simulink model "IFACS_Spring2026"  (R2025b)
settings: Solver=ode23t  StartTime=0.0  StopTime=3600*24*3  FixedStep=1  RelTol=1e-3  AbsTol=1e-3
values from neighbouring files (symbols this model uses):
  ac_cooling_capacity = 5000    [IFACS_Constants.m]
  ac_power = ac_cooling_capacity / ac_COP    (= 1250)    [IFACS_Constants.m]
  house_H = 6    [IFACS_Constants.m]
  house_L = 20    [IFACS_Constants.m]
  house_W = 10    [IFACS_Constants.m]
  roof_pitch = 15    [IFACS_Constants.m]
  TinIC = 24    [IFACS_Constants.m]
libraries: fl_lib x215, nesl_utility x52, simulink_extras x29, SimscapeFluids_lib x3
(part 1 of 5)
CloseFcn:
  | try,close(h1_HouseHeatingSystem),end
  | try,close(h2_HouseHeatingSystem),end
  | clear h1_HouseHeatingSystem h2_HouseHeatingSystem
  | 
  | clear simlog_HouseHeatingSystem
Description:
  | House Heating System
settings Model: FPTRunName=Active  ExtModeTrigMode=oneshot  ExtModeArmWhenConnect=off  ExtModeAutoUpdateStatusClock=off  VariantFading=off  Creator=The MathWorks, Inc.  LastModifiedBy=benir
settings SolverCC: AutoScaleAbsTol=off  MaxConsecutiveMinStep=10000  AlgebraicLoopSolver=TrustRegion
settings DataIOCC: ExternalInput=[]  InitialState=[]  SaveFormat=Array  SaveOutput=off  SaveTime=off  ReturnWorkspaceOutputs=off  SignalLoggingName=househeat_output
settings OptimizationCC: BlockReduction=off  BooleanDataType=off  ExpressionDepthLimit=2147483647.0  InitFltsAndDblsToZero=on  LifeSpan=inf  BufferReusableBoundary=off
settings DebuggingCC: AlgebraicLoopMsg=none  SaveWithParameterizedLinksMsg=none  SignalResolutionControl=TryResolveAllWithWarning  MultiTaskDSMMsg=warning  MultiTaskCondExecSysMsg=none  IntegerOverflowMsg=none  UnconnectedInputMsg=warning  UnconnectedOutputMsg=warning  UnconnectedLineMsg=warning  BusObjectLabelMismatch=none  AllowSymbolicDim=off  StateNameClashWarn=warning  PregeneratedLibrarySubsystemCodeDiagnostic=none  SFUnexpectedBacktrackingDiag=warning  SFNoUnconditionalDefaultTransitionDiag=warning  SFExecutionAtInitializationDiag=none  IntegerSaturationMsg=none  ArithmeticOperatorsInVariantConditions=warning
settings HardwareCC: ProdBitPerPointer=32.0  ProdBitPerSizeT=32.0  ProdBitPerPtrDiffT=32.0  ProdLargestAtomicFloat=None  ProdIntDivRoundTo=Undefined  ProdEndianess=Unspecified  ProdWordSize=32.0  ProdHWDeviceType=32-bit Generic  TargetUnknown=on
settings ModelReferenceCC: EnableRefExpFcnMdlSchedulingChecks=on  PropagateSignalLabelsOutOfModel=off
settings SFSimCC: SimUseLocalCustomCode=off  SimParseCustomCode=off  CustomCodeUndefinedFunction=UseInterfaceOnly
settings RTWCC: RTWUseLocalCustomCode=off  GPUComputeCapability=3.5  DLArmComputeVersion=19.05
settings CodeAppCC: StateflowObjectComments=on
settings GRTTargetCC: TargetFcnLib=ansi_tfl_tmw.mat  TargetLangStandard=C89/C90 (ANSI)  CombineOutputUpdateFcns=off  GRTInterface=on
settings ConfigComp: CovMetricSettings=dw  CovSaveCumulativeToWorkspaceVar=on  CovSaveSingleToWorkspaceVar=on  CovExternalEMLEnable=off  CovSFcnEnable=off
settings SimscapeCC: SimscapeLogType=all  SimscapeLogSimulationStatistics=on  SimscapeLogName=simlog_HouseHeatingSystem  SimscapeLogDataHistory=25000.0

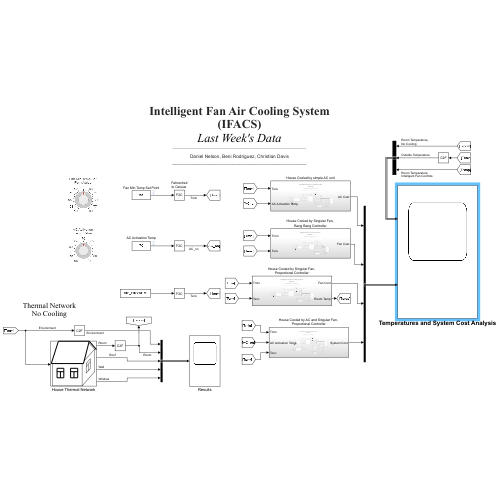
[thumbnail: Simulink's stored preview of the top-level diagram]
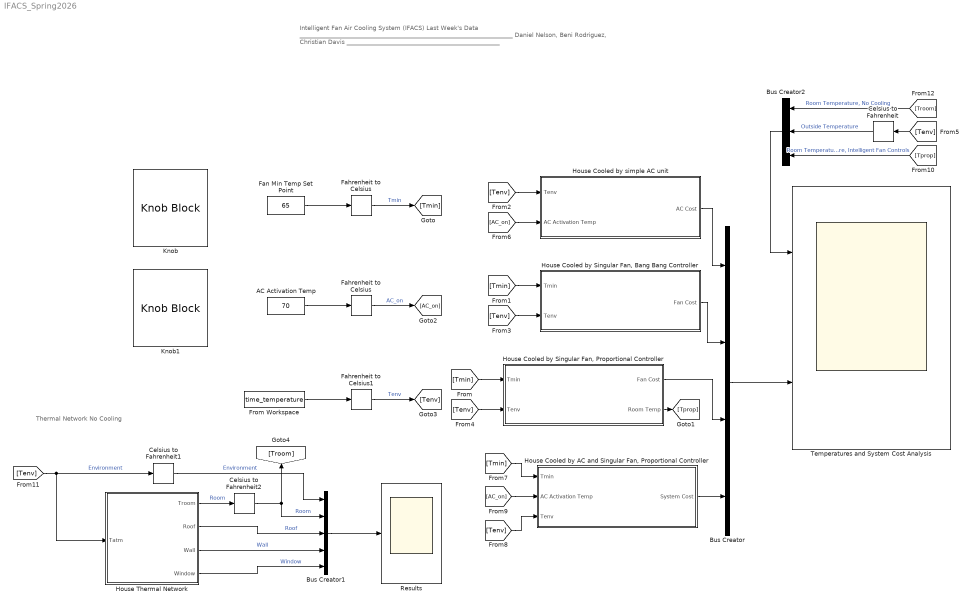
== system IFACS_Spring2026 ==
  note: Intelligent Fan Air Cooling System
      | (IFACS)
      | Last Week's Data
      | _______________________________________________________________________
      |
      | Daniel Nelson, Beni Rodriguez, Christian Davis
      | ___________________________________________________
  note: Thermal Network
      | No Cooling
  AC Activation Temp : Constant  Value=70
  Bus Creator : BusCreator  Inputs=4
  Bus Creator1 : BusCreator  Inputs=5
  Bus Creator2 : BusCreator  Inputs=3
  Celsius to Fahrenheit : simulink_extras/Transformations/Celsius to Fahrenheit
  Celsius to Fahrenheit1 : simulink_extras/Transformations/Celsius to Fahrenheit
  Celsius to Fahrenheit2 : simulink_extras/Transformations/Celsius to Fahrenheit
  Fahrenheit to Celsius : simulink_extras/Transformations/Fahrenheit to Celsius
  "Fahrenheit to Celsius " : simulink_extras/Transformations/Fahrenheit to Celsius
  Fahrenheit to Celsius1 : simulink_extras/Transformations/Fahrenheit to Celsius
  Fan Min Temp Set Point : Constant  Value=65
  From Workspace : FromWorkspace  VariableName=time_temperature
  "House Cooled by AC and Singular Fan, Proportional Controller" : Subsystem
  "House Cooled by Singular Fan, Bang Bang Controller" : Subsystem
  "House Cooled by Singular Fan, Proportional Controller" : Subsystem
  House Cooled by simple AC unit : Subsystem
  "House Thermal Network " : Subsystem  Tag=PublishSubsystem
      mask Display:
      | plot([99.4454661849886;170.309218810871;170.309218810871;99.4454661849886;99.4454661849886], [212.827470386401;212.827470386401;127.790967235342;127.790967235342;212.827470386401])
      | plot([99.4454661849886;170.309218810871], [184.481969336048;184.481969336048])
      | plot([133.460067445412;133.460067445412], [184.481969336048;127.790967235342])
      | plot([241.172971436754;312.036724062636;312.036724062636;241.172971436754;241.172971436754], [212.827470386401;212.827470386401;127.790967235342;127.790967235342;212.827470386401])
      | plot([241.172971436754;312.036724062636], [184.481969336048;184.481969336048])
      | plot([275.187572697178;275.187572697178], [184.481969336048;127.790967235342])
      | plot([113.618216710165;42.7544640842825;368.727726163343;428.253278369084], [453.764229314402;255.34572196193;255.34572196193;453.764229314402])
      | plot([428.253278369084;499.117030994967], [453.764229314402;382.900476688519])
      | plot([113.618216710165;428.253278369084], [453.764229314402;453.764229314402])
      | plot([498.86507098563;499.368991004303], [382.900476688519;382.900476688519])
      | plot([482.109730364755;496.282480889931], [382.900476688519;382.900476688519])
      | plot([482.109730364755;374.396826373413], [382.900476688519;275.187572697178])
      | plot([482.109730364755;425.418728264049], [382.900476688519;439.591478789225])
      | plot([56.927214609459;56.927214609459;354.554975638166], [255.34572196193;56.927214609459;56.927214609459])
      | plot([354.554975638166;354.554975638166], [56.927214609459;255.34572196193])
      | plot([354.554975638166;482.109730364755;482.109730364755], [56.927214609459;184.481969336048;382.900476688519])
      | plot([397.073227213696;397.073227213696;439.591478789225;439.591478789225;397.073227213696], [170.309218810871;255.34572196193;297.86397353746;209.992920281366;170.309218810871])
      | plot([397.073227213696;439.591478789225], [227.000220911577;269.518472487107])
      | plot([419.749628053978;419.749628053978], [246.842071646824;192.985619651154])
      | %patch([0;553.20969549939;553.20969549939;0;0;0.472425017505884;0.47242501750577;552.737270481884;552.737270481885;0.472425017505884;0], [496.518693398684;496.518693398684;0;0;496.518693398684;496.046268381178;0.472425017505884;0.472425017505884;496.046268381178;496.046268381178;496.518693398684], [1;1;1])
  Knob : KnobBlock  ScaleMin=50  ScaleMax=80
  Knob1 : KnobBlock  ScaleMin=50  ScaleMax=90
  Results : Scope
      settings: TimeUnits=Metric (based on Time Span)  Title=Daily Room Temp  ActiveDisplayYMinimum=61.662880384493235  ActiveDisplayYMaximum=74.086551143430853  YLabel=Temperature (F)  DataLoggingVariableName=a  DataLoggingSaveFormat=Array
  Temperatures and System Cost Analysis : Scope  NumInputPorts=2
      settings: TimeUnits=Metric (based on Time Span)  Title=Temperature  ActiveDisplayYMinimum=51.858630285523695  ActiveDisplayYMaximum=88.349041079386282  YLabel=Temperature (F)
  wires:
  Fan Min Temp Set Point/1 -> "Fahrenheit to Celsius "/1
  "Fahrenheit to Celsius "/1 -> [Tmin]  "Tmin"
  [Tenv] -> House Cooled by simple AC unit/1(Tenv)
  [Tmin] -> "House Cooled by Singular Fan, Bang Bang Controller"/1(Tmin)
  [Tenv] -> "House Cooled by Singular Fan, Bang Bang Controller"/2(Tenv)
  "House Cooled by Singular Fan, Proportional Controller"/1(Fan Cost) -> Bus Creator/3
  "House Cooled by Singular Fan, Bang Bang Controller"/1(Fan Cost) -> Bus Creator/2
  House Cooled by simple AC unit/1(AC Cost) -> Bus Creator/1
  [Tenv] -> Celsius to Fahrenheit/1
  AC Activation Temp/1 -> Fahrenheit to Celsius/1
  Fahrenheit to Celsius/1 -> [AC_on]  "AC_on"
  [AC_on] -> House Cooled by simple AC unit/2(AC Activation Temp)
  From Workspace/1 -> Fahrenheit to Celsius1/1
  [Tmin] -> "House Cooled by AC and Singular Fan, Proportional Controller"/1(Tmin)
  [Tenv] -> "House Cooled by AC and Singular Fan, Proportional Controller"/3(Tenv)
  [AC_on] -> "House Cooled by AC and Singular Fan, Proportional Controller"/2(AC Activation Temp)
  "House Cooled by AC and Singular Fan, Proportional Controller"/1(System Cost) -> Bus Creator/4
  Fahrenheit to Celsius1/1 -> [Tenv]  "Tenv"
  Bus Creator/1 -> Temperatures and System Cost Analysis/2
  [Tprop] -> Bus Creator2/3  "Room Temperature, Intelligent Fan Controls"
  Celsius to Fahrenheit/1 -> Bus Creator2/2  "Outside Temperature"
  Bus Creator2/1 -> Temperatures and System Cost Analysis/1
  "House Cooled by Singular Fan, Proportional Controller"/2(Room Temp) -> [Tprop]
  [Tmin] -> "House Cooled by Singular Fan, Proportional Controller"/1(Tmin)
  [Tenv] -> "House Cooled by Singular Fan, Proportional Controller"/2(Tenv)
  "House Thermal Network "/4(Window) -> Bus Creator1/5  "Window"
  "House Thermal Network "/3(Wall) -> Bus Creator1/4  "Wall"
  Celsius to Fahrenheit1/1 -> Bus Creator1/1  "Environment"
  Bus Creator1/1 -> Results/1
  "House Thermal Network "/1(Troom) -> Celsius to Fahrenheit2/1  "Room"
  "House Thermal Network "/2(Roof) -> Bus Creator1/3  "Roof"
  [Tenv] -> "House Thermal Network "/1(Tatm), Celsius to Fahrenheit1/1  "Environment"
  Celsius to Fahrenheit2/1 -> [Troom], Bus Creator1/2  "Room"
  [Troom] -> Bus Creator2/1  "Room Temperature, No Cooling"

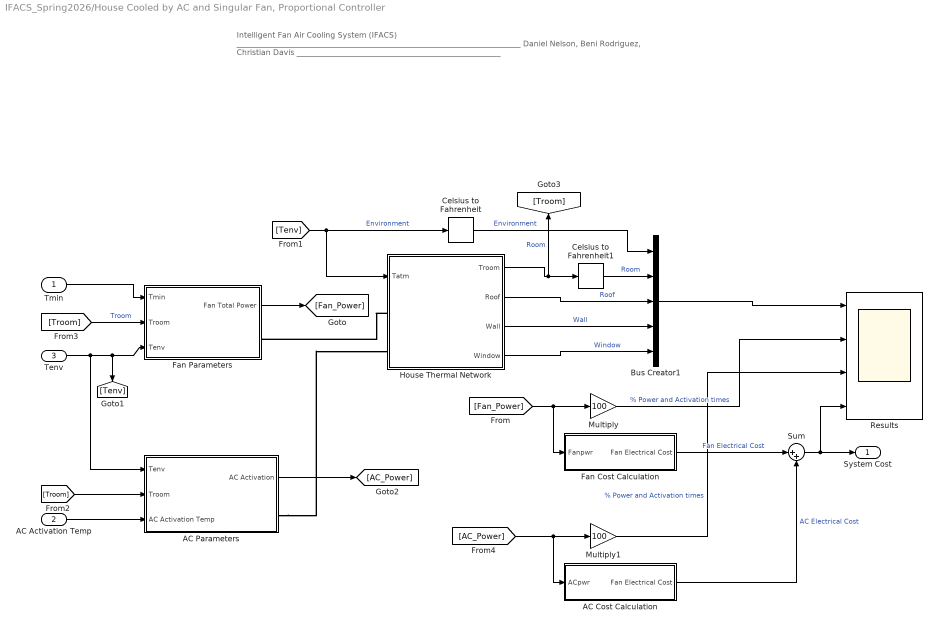
== system IFACS_Spring2026/House Cooled by AC and Singular Fan, Proportional Controller ==
  note: Intelligent Fan Air Cooling System
      | (IFACS)
      | _______________________________________________________________________
      |
      | Daniel Nelson, Beni Rodriguez, Christian Davis
      | ___________________________________________________
  Tmin : Inport
  AC Activation Temp : Inport  Port=2
  Tenv : Inport  Port=3
  AC Cost Calculation : Subsystem
  AC Parameters : Subsystem
  Bus Creator1 : BusCreator  Inputs=5
  Celsius to Fahrenheit : simulink_extras/Transformations/Celsius to Fahrenheit
  Celsius to Fahrenheit1 : simulink_extras/Transformations/Celsius to Fahrenheit
  Fan Cost Calculation : Subsystem
  Fan Parameters : Subsystem
  House Thermal Network : Subsystem  Tag=PublishSubsystem
      mask Display:
      | plot([99.4454661849886;170.309218810871;170.309218810871;99.4454661849886;99.4454661849886], [212.827470386401;212.827470386401;127.790967235342;127.790967235342;212.827470386401])
      | plot([99.4454661849886;170.309218810871], [184.481969336048;184.481969336048])
      | plot([133.460067445412;133.460067445412], [184.481969336048;127.790967235342])
      | plot([241.172971436754;312.036724062636;312.036724062636;241.172971436754;241.172971436754], [212.827470386401;212.827470386401;127.790967235342;127.790967235342;212.827470386401])
      | plot([241.172971436754;312.036724062636], [184.481969336048;184.481969336048])
      | plot([275.187572697178;275.187572697178], [184.481969336048;127.790967235342])
      | plot([113.618216710165;42.7544640842825;368.727726163343;428.253278369084], [453.764229314402;255.34572196193;255.34572196193;453.764229314402])
      | plot([428.253278369084;499.117030994967], [453.764229314402;382.900476688519])
      | plot([113.618216710165;428.253278369084], [453.764229314402;453.764229314402])
      | plot([498.86507098563;499.368991004303], [382.900476688519;382.900476688519])
      | plot([482.109730364755;496.282480889931], [382.900476688519;382.900476688519])
      | plot([482.109730364755;374.396826373413], [382.900476688519;275.187572697178])
      | plot([482.109730364755;425.418728264049], [382.900476688519;439.591478789225])
      | plot([56.927214609459;56.927214609459;354.554975638166], [255.34572196193;56.927214609459;56.927214609459])
      | plot([354.554975638166;354.554975638166], [56.927214609459;255.34572196193])
      | plot([354.554975638166;482.109730364755;482.109730364755], [56.927214609459;184.481969336048;382.900476688519])
      | plot([397.073227213696;397.073227213696;439.591478789225;439.591478789225;397.073227213696], [170.309218810871;255.34572196193;297.86397353746;209.992920281366;170.309218810871])
      | plot([397.073227213696;439.591478789225], [227.000220911577;269.518472487107])
      | plot([419.749628053978;419.749628053978], [246.842071646824;192.985619651154])
      | %patch([0;553.20969549939;553.20969549939;0;0;0.472425017505884;0.47242501750577;552.737270481884;552.737270481885;0.472425017505884;0], [496.518693398684;496.518693398684;0;0;496.518693398684;496.046268381178;0.472425017505884;0.472425017505884;496.046268381178;496.046268381178;496.518693398684], [1;1;1])
  Multiply : Gain  Gain=100
  Multiply1 : Gain  Gain=100
  Results : Scope  NumInputPorts=4
      settings: TimeUnits=Metric (based on Time Span)  ActiveDisplayString=4  Title=Total System Cost  ActiveDisplayYMinimum=-0.28869506365036945  ActiveDisplayYMaximum=5.4852062093570213  YLabel=System Cost ($)  DataLoggingVariableName=a3  DataLoggingSaveFormat=Array
  Sum : Sum  Inputs=|++
  System Cost : Outport
  wires:
  Bus Creator1/1 -> Results/1
  [Tenv] -> House Thermal Network/1(Tatm), Celsius to Fahrenheit/1  "Environment"
  House Thermal Network/1(Troom) -> Celsius to Fahrenheit1/1, [Troom]  "Room"
  Multiply/1 -> Results/2  "% Power and Activation times"
  House Thermal Network/2(Roof) -> Bus Creator1/3  "Roof"
  House Thermal Network/3(Wall) -> Bus Creator1/4  "Wall"
  House Thermal Network/4(Window) -> Bus Creator1/5  "Window"
  Tenv/1 -> AC Parameters/1(Tenv), Fan Parameters/3(Tenv), [Tenv]
  [Fan_Power] -> Fan Cost Calculation/1(Fanpwr), Multiply/1
  Celsius to Fahrenheit1/1 -> Bus Creator1/2  "Room"
  Celsius to Fahrenheit/1 -> Bus Creator1/1  "Environment"
  Tmin/1 -> Fan Parameters/1(Tmin)
  [Troom] -> Fan Parameters/2(Troom)  "Troom"
  Fan Parameters/1(Fan Total Power) -> [Fan_Power]
  Fan Cost Calculation/1(Fan Electrical Cost) -> Sum/1  "Fan Electrical Cost"
  AC Activation Temp/1 -> AC Parameters/3(AC Activation Temp)
  [Troom] -> AC Parameters/2(Troom)
  Multiply1/1 -> Results/3  "% Power and Activation times"
  AC Cost Calculation/1(Fan Electrical Cost) -> Sum/2  "AC Electrical Cost"
  [AC_Power] -> AC Cost Calculation/1(ACpwr), Multiply1/1
  Sum/1 -> Results/4, System Cost/1
  AC Parameters/1(AC Activation) -> [AC_Power]
  connections:
  House Thermal Network/LConn1 -- Fan Parameters/RConn1
  AC Parameters/RConn1 -- House Thermal Network/LConn2

== system IFACS_Spring2026/House Cooled by Singular Fan, Bang Bang Controller ==
  note: Intelligent Fan Air Cooling System
      | (IFACS)
      | _______________________________________________________________________
      |
      | Daniel Nelson, Beni Rodriguez, Christian Davis
      | ___________________________________________________
  Tmin : Inport
  Tenv : Inport  Port=2
  Bus Creator1 : BusCreator  Inputs=5
  Celsius to Fahrenheit : simulink_extras/Transformations/Celsius to Fahrenheit
  Celsius to Fahrenheit1 : simulink_extras/Transformations/Celsius to Fahrenheit
  Fan Cost Calculation : Subsystem
  Fan Parameters : Subsystem
  House Thermal Network : Subsystem  Tag=PublishSubsystem
      mask Display:
      | plot([99.4454661849886;170.309218810871;170.309218810871;99.4454661849886;99.4454661849886], [212.827470386401;212.827470386401;127.790967235342;127.790967235342;212.827470386401])
      | plot([99.4454661849886;170.309218810871], [184.481969336048;184.481969336048])
      | plot([133.460067445412;133.460067445412], [184.481969336048;127.790967235342])
      | plot([241.172971436754;312.036724062636;312.036724062636;241.172971436754;241.172971436754], [212.827470386401;212.827470386401;127.790967235342;127.790967235342;212.827470386401])
      | plot([241.172971436754;312.036724062636], [184.481969336048;184.481969336048])
      | plot([275.187572697178;275.187572697178], [184.481969336048;127.790967235342])
      | plot([113.618216710165;42.7544640842825;368.727726163343;428.253278369084], [453.764229314402;255.34572196193;255.34572196193;453.764229314402])
      | plot([428.253278369084;499.117030994967], [453.764229314402;382.900476688519])
      | plot([113.618216710165;428.253278369084], [453.764229314402;453.764229314402])
      | plot([498.86507098563;499.368991004303], [382.900476688519;382.900476688519])
      | plot([482.109730364755;496.282480889931], [382.900476688519;382.900476688519])
      | plot([482.109730364755;374.396826373413], [382.900476688519;275.187572697178])
      | plot([482.109730364755;425.418728264049], [382.900476688519;439.591478789225])
      | plot([56.927214609459;56.927214609459;354.554975638166], [255.34572196193;56.927214609459;56.927214609459])
      | plot([354.554975638166;354.554975638166], [56.927214609459;255.34572196193])
      | plot([354.554975638166;482.109730364755;482.109730364755], [56.927214609459;184.481969336048;382.900476688519])
      | plot([397.073227213696;397.073227213696;439.591478789225;439.591478789225;397.073227213696], [170.309218810871;255.34572196193;297.86397353746;209.992920281366;170.309218810871])
      | plot([397.073227213696;439.591478789225], [227.000220911577;269.518472487107])
      | plot([419.749628053978;419.749628053978], [246.842071646824;192.985619651154])
      | %patch([0;553.20969549939;553.20969549939;0;0;0.472425017505884;0.47242501750577;552.737270481884;552.737270481885;0.472425017505884;0], [496.518693398684;496.518693398684;0;0;496.518693398684;496.046268381178;0.472425017505884;0.472425017505884;496.046268381178;496.046268381178;496.518693398684], [1;1;1])
  Multiply : Gain  Gain=100
  Results : Scope  NumInputPorts=3
      settings: TimeUnits=Metric (based on Time Span)  ActiveDisplayString=3  Title=Fan Cost  ActiveDisplayYMinimum=-0.053943140725414111  ActiveDisplayYMaximum=0.48548826652872712  YLabel=Fan Cost ($)  DataLoggingVariableName=a3  DataLoggingSaveFormat=Array
  Fan Cost : Outport
  wires:
  Bus Creator1/1 -> Results/1
  [Tenv] -> House Thermal Network/1(Tatm), Celsius to Fahrenheit/1  "Environment"
  House Thermal Network/1(Troom) -> Celsius to Fahrenheit1/1, [Troom]  "Room"
  Multiply/1 -> Results/2  "% Power and Activation times"
  House Thermal Network/3(Wall) -> Bus Creator1/4  "Wall"
  House Thermal Network/4(Window) -> Bus Creator1/5  "Window"
  Tenv/1 -> Fan Parameters/3(Tenv), [Tenv]
  [Fan_Power] -> Fan Cost Calculation/1(Fanpwr), Multiply/1
  Celsius to Fahrenheit1/1 -> Bus Creator1/2  "Room"
  Celsius to Fahrenheit/1 -> Bus Creator1/1  "Environment"
  Tmin/1 -> Fan Parameters/1(Tmin)
  [Troom] -> Fan Parameters/2(Troom)  "Troom"
  Fan Parameters/1(Fan Total Power) -> [Fan_Power]
  House Thermal Network/2(Roof) -> Bus Creator1/3  "Roof"
  Fan Cost Calculation/1(Fan Electrical Cost) -> Results/3, Fan Cost/1  "Fan Electrical Cost"
  connections:
  House Thermal Network/LConn1 -- Fan Parameters/RConn1

== system IFACS_Spring2026/House Cooled by Singular Fan, Proportional Controller ==
  note: Intelligent Fan Air Cooling System
      | (IFACS)
      | _______________________________________________________________________
      |
      | Daniel Nelson, Beni Rodriguez, Christian Davis
      | ___________________________________________________
  Tmin : Inport
  Tenv : Inport  Port=2
  Bus Creator1 : BusCreator  Inputs=5
  Celsius to Fahrenheit : simulink_extras/Transformations/Celsius to Fahrenheit
  Celsius to Fahrenheit1 : simulink_extras/Transformations/Celsius to Fahrenheit
  Fan Cost Calculation : Subsystem
  Fan Parameters : Subsystem
  House Thermal Network : Subsystem  Tag=PublishSubsystem
      mask Display:
      | plot([99.4454661849886;170.309218810871;170.309218810871;99.4454661849886;99.4454661849886], [212.827470386401;212.827470386401;127.790967235342;127.790967235342;212.827470386401])
      | plot([99.4454661849886;170.309218810871], [184.481969336048;184.481969336048])
      | plot([133.460067445412;133.460067445412], [184.481969336048;127.790967235342])
      | plot([241.172971436754;312.036724062636;312.036724062636;241.172971436754;241.172971436754], [212.827470386401;212.827470386401;127.790967235342;127.790967235342;212.827470386401])
      | plot([241.172971436754;312.036724062636], [184.481969336048;184.481969336048])
      | plot([275.187572697178;275.187572697178], [184.481969336048;127.790967235342])
      | plot([113.618216710165;42.7544640842825;368.727726163343;428.253278369084], [453.764229314402;255.34572196193;255.34572196193;453.764229314402])
      | plot([428.253278369084;499.117030994967], [453.764229314402;382.900476688519])
      | plot([113.618216710165;428.253278369084], [453.764229314402;453.764229314402])
      | plot([498.86507098563;499.368991004303], [382.900476688519;382.900476688519])
      | plot([482.109730364755;496.282480889931], [382.900476688519;382.900476688519])
      | plot([482.109730364755;374.396826373413], [382.900476688519;275.187572697178])
      | plot([482.109730364755;425.418728264049], [382.900476688519;439.591478789225])
      | plot([56.927214609459;56.927214609459;354.554975638166], [255.34572196193;56.927214609459;56.927214609459])
      | plot([354.554975638166;354.554975638166], [56.927214609459;255.34572196193])
      | plot([354.554975638166;482.109730364755;482.109730364755], [56.927214609459;184.481969336048;382.900476688519])
      | plot([397.073227213696;397.073227213696;439.591478789225;439.591478789225;397.073227213696], [170.309218810871;255.34572196193;297.86397353746;209.992920281366;170.309218810871])
      | plot([397.073227213696;439.591478789225], [227.000220911577;269.518472487107])
      | plot([419.749628053978;419.749628053978], [246.842071646824;192.985619651154])
      | %patch([0;553.20969549939;553.20969549939;0;0;0.472425017505884;0.47242501750577;552.737270481884;552.737270481885;0.472425017505884;0], [496.518693398684;496.518693398684;0;0;496.518693398684;496.046268381178;0.472425017505884;0.472425017505884;496.046268381178;496.046268381178;496.518693398684], [1;1;1])
  Multiply : Gain  Gain=100
  Results : Scope  NumInputPorts=3
      settings: TimeUnits=Metric (based on Time Span)  Title=Fan Power  ActiveDisplayYMinimum=-11.770479028172618  ActiveDisplayYMaximum=105.93431125355357  YLabel=Fan Power (%)  DataLoggingVariableName=a3  DataLoggingSaveFormat=Array
  Fan Cost : Outport
  Room Temp : Outport  Port=2
  wires:
  Bus Creator1/1 -> Results/1
  [Tenv] -> House Thermal Network/1(Tatm), Celsius to Fahrenheit/1  "Environment"
  House Thermal Network/1(Troom) -> Celsius to Fahrenheit1/1, [Troom]  "Room"
  Multiply/1 -> Results/2  "% Power and Activation times"
  House Thermal Network/2(Roof) -> Bus Creator1/3  "Roof"
  House Thermal Network/3(Wall) -> Bus Creator1/4  "Wall"
  House Thermal Network/4(Window) -> Bus Creator1/5  "Window"
  Tenv/1 -> Fan Parameters/3(Tenv), [Tenv]
  [Fan_Power] -> Fan Cost Calculation/1(Fanpwr), Multiply/1
  Celsius to Fahrenheit1/1 -> Room Temp/1, Bus Creator1/2  "Room"
  Celsius to Fahrenheit/1 -> Bus Creator1/1  "Environment"
  Tmin/1 -> Fan Parameters/1(Tmin)
  [Troom] -> Fan Parameters/2(Troom)  "Troom"
  Fan Parameters/1(Fan Total Power) -> [Fan_Power]
  Fan Cost Calculation/1(Fan Electrical Cost) -> Results/3, Fan Cost/1  "Fan Electrical Cost"
  connections:
  House Thermal Network/LConn1 -- Fan Parameters/RConn1

== system IFACS_Spring2026/House Cooled by simple AC unit ==
  note: Intelligent Fan Air Cooling System
      | (IFACS)
      | _______________________________________________________________________
      |
      | Daniel Nelson, Beni Rodriguez, Christian Davis
      | ___________________________________________________
  Tenv : Inport
  AC Activation Temp : Inport  Port=2
  AC Cost Calculation : Subsystem
  AC Parameters : Subsystem
  Bus Creator1 : BusCreator  Inputs=5
  Celsius to Fahrenheit : simulink_extras/Transformations/Celsius to Fahrenheit
  Celsius to Fahrenheit1 : simulink_extras/Transformations/Celsius to Fahrenheit
  House Thermal Network : Subsystem  Tag=PublishSubsystem
      mask Display:
      | plot([99.4454661849886;170.309218810871;170.309218810871;99.4454661849886;99.4454661849886], [212.827470386401;212.827470386401;127.790967235342;127.790967235342;212.827470386401])
      | plot([99.4454661849886;170.309218810871], [184.481969336048;184.481969336048])
      | plot([133.460067445412;133.460067445412], [184.481969336048;127.790967235342])
      | plot([241.172971436754;312.036724062636;312.036724062636;241.172971436754;241.172971436754], [212.827470386401;212.827470386401;127.790967235342;127.790967235342;212.827470386401])
      | plot([241.172971436754;312.036724062636], [184.481969336048;184.481969336048])
      | plot([275.187572697178;275.187572697178], [184.481969336048;127.790967235342])
      | plot([113.618216710165;42.7544640842825;368.727726163343;428.253278369084], [453.764229314402;255.34572196193;255.34572196193;453.764229314402])
      | plot([428.253278369084;499.117030994967], [453.764229314402;382.900476688519])
      | plot([113.618216710165;428.253278369084], [453.764229314402;453.764229314402])
      | plot([498.86507098563;499.368991004303], [382.900476688519;382.900476688519])
      | plot([482.109730364755;496.282480889931], [382.900476688519;382.900476688519])
      | plot([482.109730364755;374.396826373413], [382.900476688519;275.187572697178])
      | plot([482.109730364755;425.418728264049], [382.900476688519;439.591478789225])
      | plot([56.927214609459;56.927214609459;354.554975638166], [255.34572196193;56.927214609459;56.927214609459])
      | plot([354.554975638166;354.554975638166], [56.927214609459;255.34572196193])
      | plot([354.554975638166;482.109730364755;482.109730364755], [56.927214609459;184.481969336048;382.900476688519])
      | plot([397.073227213696;397.073227213696;439.591478789225;439.591478789225;397.073227213696], [170.309218810871;255.34572196193;297.86397353746;209.992920281366;170.309218810871])
      | plot([397.073227213696;439.591478789225], [227.000220911577;269.518472487107])
      | plot([419.749628053978;419.749628053978], [246.842071646824;192.985619651154])
      | %patch([0;553.20969549939;553.20969549939;0;0;0.472425017505884;0.47242501750577;552.737270481884;552.737270481885;0.472425017505884;0], [496.518693398684;496.518693398684;0;0;496.518693398684;496.046268381178;0.472425017505884;0.472425017505884;496.046268381178;496.046268381178;496.518693398684], [1;1;1])
  Multiply : Gain  Gain=100
  Results : Scope  NumInputPorts=3
      settings: TimeUnits=Metric (based on Time Span)  ActiveDisplayString=3  ActiveDisplayYMinimum=-0.20049406109345627  ActiveDisplayYMaximum=1.8044465498411069  YLabel=AC Cost ($)  DataLoggingVariableName=a3  DataLoggingSaveFormat=Array
  AC Cost : Outport
  wires:
  Bus Creator1/1 -> Results/1
  [Tenv] -> House Thermal Network/1(Tatm), Celsius to Fahrenheit/1  "Environment"
  House Thermal Network/1(Troom) -> Celsius to Fahrenheit1/1, [Troom]  "Room"
  Multiply/1 -> Results/2  "% Power and Activation times"
  House Thermal Network/2(Roof) -> Bus Creator1/3  "Roof"
  House Thermal Network/3(Wall) -> Bus Creator1/4  "Wall"
  House Thermal Network/4(Window) -> Bus Creator1/5  "Window"
  Tenv/1 -> AC Parameters/3(Tenv), [Tenv]
  [AC_Power] -> AC Cost Calculation/1(ACpwr), Multiply/1
  Celsius to Fahrenheit1/1 -> Bus Creator1/2  "Room"
  Celsius to Fahrenheit/1 -> Bus Creator1/1  "Environment"
  [Troom] -> AC Parameters/1(Troom)  "Troom"
  AC Parameters/1(AC Activation) -> [AC_Power]
  AC Cost Calculation/1(Fan Electrical Cost) -> Results/3, AC Cost/1  "AC Electrical Cost"
  AC Activation Temp/1 -> AC Parameters/2(AC Activation Temp)
  connections:
  House Thermal Network/LConn1 -- AC Parameters/RConn1

== system IFACS_Spring2026/House Thermal Network  ==
  Tatm : Inport
  Controlled Temperature Source : fl_lib/Thermal/Thermal Sources/Controlled Temperature Source
  House Thermal Network : Subsystem  Tag=PublishSubsystem  mask(House Thermal Network){area_roof=2 * house_L * house_W / (2*cosd(roof_pitch)), thickness_roof=0.2, rho_roof=32, cp_roof=835, k_roof=0.038, hc_roof_interior=12, hc_roof_exterior=38, T_init_roof=TinIC, area_wall=2 * (house_L + house_W) * house_H, thickness_wall=0.2, rho_wall=1920, cp_wall=835, k_wall=0.038, hc_wall_interior=24, hc_wall_exterior=34, T_init_wall=TinIC, area_wall_inside=(house_L + 2 * house_W) * house_H + 2 * house_L * house_W, thickness_wall_inside=0.15, rho_wall_inside=10, cp_wall_inside=1000, k_wall_inside=0.2, hc_wall_inside_interior=24, T_init_wall_inside=TinIC, area_window=12, thickness_window=0.01, rho_window=2700, cp_window=840, k_window=0.78, hc_window_interior=25, hc_window_exterior=32, T_init_window=TinIC, area_furniture=300, M_furniture=3000, cp_furniture=2000, hc_furniture_interior=18, T_init_furniture=TinIC}
      mask prompts: area_roof "Total area (m^2)"; thickness_roof "Average thickness (m)"; rho_roof "Average density (kg/m^3)"; cp_roof "Average specific heat (J/kg/K)"; k_roof "Average conductivity (W/m/K)"; hc_roof_interior "Interior heat transfer coefficient (W/m^2/K)"; hc_roof_exterior "Exterior heat transfer coefficient (W/m^2/K)"; T_init_roof "Initial temperature (degC)"; area_wall "Total area (m^2)"; thickness_wall "Average thickness (m)"; rho_wall "Average density (kg/m^3)"; cp_wall "Average specific heat (J/kg/K)"; k_wall "Average conductivity (W/m/K)"; hc_wall_interior "Interior heat transfer coefficient (W/m^2/K)"; hc_wall_exterior "Exterior heat transfer coefficient (W/m^2/K)"; T_init_wall "Initial temperature (degC)"; area_wall_inside "Total area (m^2)"; thickness_wall_inside "Average thickness (m)"; rho_wall_inside "Average density (kg/m^3)"; cp_wall_inside "Average specific heat (J/kg/K)"; k_wall_inside "Average conductivity (W/m/K)"; hc_wall_inside_interior "Interior heat transfer coefficient (W/m^2/K)"; T_init_wall_inside "Initial temperature (degC)"; area_window "Total area (m^2)"; thickness_window "Average thickness (m)"; rho_window "Average density (kg/m^3)"; cp_window "Average specific heat (J/kg/K)"; k_window "Average conductivity (W/m/K)"; hc_window_interior "Interior heat transfer coefficient (W/m^2/K)"; hc_window_exterior "Exterior heat transfer coefficient (W/m^2/K)"; T_init_window "Initial temperature (degC)"; area_furniture "Total surface area (m^2)"; M_furniture "Total mass (kg)"; cp_furniture "Average specific heat (J/kg/K)"; hc_furniture_interior "Interior heat transfer coefficient (W/m^2/K)"; T_init_furniture "Initial temperature (degC)"
      mask help: This subsystem models heat transfer between the air in the interior of the house and the external environment.
      mask DialogControl TabRoof Prompt: Roof
      mask DialogControl TabWall Prompt: Exterior Walls
      mask DialogControl TabWallInside Prompt: Interior Walls
      mask DialogControl TabWindow Prompt: Windows
      mask DialogControl TabFurniture Prompt: Furniture
  PS2S : nesl_utility/PS-Simulink Converter  PhysicalDomain=network_engine_domain  SubClassName=ps_output  LeftPortType=input  RightPortType=output  PseudoPeriodic=off  Frequencies=[]  VectorFormat=1-D array  Unit=degC  AffineConversion=on
  Simulink-PS Converter : nesl_utility/Simulink-PS Converter  PhysicalDomain=network_engine_domain  SubClassName=ps_input  LeftPortType=input  RightPortType=output  PseudoPeriodic=off  Frequencies=[]  NoiseDistribution=none  NoiseParameters=[]  Unit=degC  AffineConversion=on  FilteringAndDerivatives=zero  SimscapeFilterOrder=1  InputFilterTimeConstant=.001  UdotUserProvided=0
  Solver Configuration : nesl_utility/Solver Configuration  PhysicalDomain=network_engine_domain  SubClassName=solver  LeftPortType=input  RightPortType=generic  Tones=[]  Harmonics=[]  SimulateNoise=off  Profile=off  UseLocalSampling=off  EnableSwitchedLinearOptims=on  FrequencyDomain=off  UseCCode=off  RelTol=0.001  AbsTol=1e-06  MinStep=1e-09  ToWorkspace=off  RevertToSquareIcSolve=off  NumHomotopyIterations=100  PhasorMode=off  PhasorModeNumHarmonics=1  ConsistencySolver=NEWTON_XTOL_AFTER_FTOL  IndexReductionMethod=DerivativeReplacement  DoDC=off  ResidualTolerance=1e-9  ConsistencyTolSource=GLOBAL  ConsistencyAbsTol=0.001  ConsistencyRelTol=0.001  ConsistencyTolFactor=0.001  UseLocalSolver=off  LocalSolverChoice=NE_BACKWARD_EULER_ADVANCER  ResolveIndetEquations=on  FunctionEvalNumThread=1  LocalSolverSampleTime=1  DoFixedCost=off  MaxNonlinIter=3  MaxModeIter=2  ComputeImpulses=off  ImpulseIterations=2  LinearAlgebra=auto  LinearAlgebraNumThread=0  EquationFormulation=NE_TIME_EF  DelaysMemoryBudget=1024  AutomaticFiltering=on  FilteringTimeConstant=0.001  PartitionStorageMethod=AS_NEEDED  PartitionMemoryBudget=1024  PartitionMethod=FAST  MultibodyUseLocalSolver=off  MultibodyLocalSolverChoice=ODE1  MultibodyLocalSolverSampleTime=0.001
  TRef : fl_lib/Thermal/Thermal Elements/Thermal Reference
  Temperature Sensor : fl_lib/Thermal/Thermal Sensors/Temperature Sensor  temperature_measure=foundation.enum.MeasurementReference.difference
  Thermal Mass Air : fl_lib/Thermal/Thermal Elements/Thermal Mass  mass_type=foundation.enum.constant_variable.constant  mass=1600 kg  sp_heat=c_air J/kg/K  mass_min=1e-6 kg  num_ports=foundation.enum.numPorts2.one  m_specify=off  m_priority=High  m=1 kg  m_nominal_specify=off  m_nominal_value=1  m_nominal_unit=kg  T_specify=on  T_priority=High  T=TinIC degC  T_nominal_specify=off  T_nominal_value=1  T_nominal_unit=K  Q_specify=off  Q_priority=None  Q=0 W  Q_nominal_specify=off  Q_nominal_value=1  Q_nominal_unit=W
  Thermal Reference : fl_lib/Thermal/Thermal Elements/Thermal Reference
  Troom : Outport  VectorParamsAs1DForOutWhenUnconnected=off
  Roof : Outport  Port=2  VectorParamsAs1DForOutWhenUnconnected=off
  Wall : Outport  Port=3  VectorParamsAs1DForOutWhenUnconnected=off
  Window : Outport  Port=4  VectorParamsAs1DForOutWhenUnconnected=off
  wires:
  Tatm/1 -> Simulink-PS Converter/1
  House Thermal Network/1(Roof) -> [Roof]
  [Roof] -> Roof/1
  House Thermal Network/2(Wall) -> [Wall]
  [Wall] -> Wall/1
  House Thermal Network/3(Window) -> [Window]
  [Window] -> Window/1
  PS2S/1 -> Troom/1  "Room"
  connections:
  Thermal Reference/LConn1 -- Controlled Temperature Source/RConn2
  Solver Configuration/RConn1 -- Simulink-PS Converter/RConn1 -- Controlled Temperature Source/RConn1
  Thermal Mass Air/LConn1 -- House Thermal Network/RConn1 -- Temperature Sensor/LConn1
  Temperature Sensor/RConn1 -- TRef/LConn1
  PS2S/LConn1 -- Temperature Sensor/RConn2
  House Thermal Network/LConn1 -- Controlled Temperature Source/LConn1

== system IFACS_Spring2026/House Cooled by AC and Singular Fan, Proportional Controller/AC Cost Calculation ==
  ACpwr : Inport
  Electricity Cost (per kWh) : Gain  Gain=.15
  Fan Wattage : Gain  Gain=ac_power/(1000*3600)
  Integrator : Integrator
  Fan Electrical Cost : Outport
  wires:
  Electricity Cost (per kWh)/1 -> Fan Electrical Cost/1  "Fan Electricity Cost"
  Integrator/1 -> Fan Wattage/1
  Fan Wattage/1 -> Electricity Cost (per kWh)/1
  ACpwr/1 -> Integrator/1

== system IFACS_Spring2026/House Cooled by AC and Singular Fan, Proportional Controller/AC Parameters ==
  Tenv : Inport
  Troom : Inport  Port=2
  AC Activation Temp : Inport  Port=3
  ACEnable : Product  Inputs=**
  CoolingSrc : fl_lib/Thermal/Thermal Sources/Controlled Heat Flow Rate Source
  OutdoorWarm : Relay  OnSwitchValue=.0001  OffSwitchValue=-2
  Qac_Scale : Gain  Gain=-ac_cooling_capacity
  S2PS_Qac : nesl_utility/Simulink-PS Converter  PhysicalDomain=network_engine_domain  SubClassName=ps_input  LeftPortType=input  RightPortType=output  PseudoPeriodic=off  Frequencies=[]  NoiseDistribution=none  NoiseParameters=[]  Unit=W  AffineConversion=off  FilteringAndDerivatives=provide  SimscapeFilterOrder=1  InputFilterTimeConstant=0.001  UdotUserProvided=0
  Sum : Sum  Inputs=|+-
  Sum1 : Sum  Inputs=|+-
  TRef : fl_lib/Thermal/Thermal Elements/Thermal Reference
  TooHot : Relay  OnSwitchValue=.0001  OffSwitchValue=-1
  AC Output : PMIOPort  Side=Right
  AC Activation : Outport
  wires:
  OutdoorWarm/1 -> ACEnable/2
  TooHot/1 -> ACEnable/1
  ACEnable/1 -> AC Activation/1, Qac_Scale/1
  Qac_Scale/1 -> S2PS_Qac/1
  Tenv/1 -> Sum1/1
  Sum1/1 -> OutdoorWarm/1
  Sum/1 -> TooHot/1
  AC Activation Temp/1 -> Sum/2, Sum1/2
  Troom/1 -> Sum/1
  connections:
  AC Output/RConn1 -- CoolingSrc/LConn1
  S2PS_Qac/RConn1 -- CoolingSrc/RConn1
  TRef/LConn1 -- CoolingSrc/RConn2

== system IFACS_Spring2026/House Cooled by AC and Singular Fan, Proportional Controller/Fan Cost Calculation ==
  Fanpwr : Inport
  Electricity Cost (per kWh) : Gain  Gain=.15
  Fan Wattage : Gain  Gain=68.9/(1000*3600)
  Integrator : Integrator
  Fan Electrical Cost : Outport
  wires:
  Electricity Cost (per kWh)/1 -> Fan Electrical Cost/1  "Fan Electricity Cost"
  Integrator/1 -> Fan Wattage/1
  Fan Wattage/1 -> Electricity Cost (per kWh)/1
  Fanpwr/1 -> Integrator/1

== system IFACS_Spring2026/House Cooled by AC and Singular Fan, Proportional Controller/Fan Parameters ==
  note: Current Fan used in Simulation
      | https://www.homedepot.com/p/KIWDZFU-720-CFM-Wall-Mounted-Ventilation-Fan-for-Home-Garage-and-Office-Use-423D22SA17036/335970250?MERCH=REC-_-brand_based_collection-_-335970202-_-3-_-n/a-_-n/a-_-n/a-_-n/a-_-n/a
  Tmin : Inport
  Troom : Inport  Port=2
  Tenv : Inport  Port=3
  Fan Activation : Subsystem
  House Fan : Subsystem
  Fan Output : PMIOPort  Side=Right
  Fan Total Power : Outport
  wires:
  Fan Activation/1(Fan Activation) -> House Fan/1(Fan Activation)
  Tmin/1 -> Fan Activation/1(Tmin)
  Fan Activation/2(Fan Power) -> House Fan/2(Fan Power)
  Tenv/1 -> Fan Activation/3(Tenv), House Fan/3(Tenv)
  House Fan/1(Fan Total Power) -> Fan Total Power/1
  Troom/1 -> Fan Activation/2(Room)
  connections:
  Fan Output/RConn1 -- House Fan/RConn1

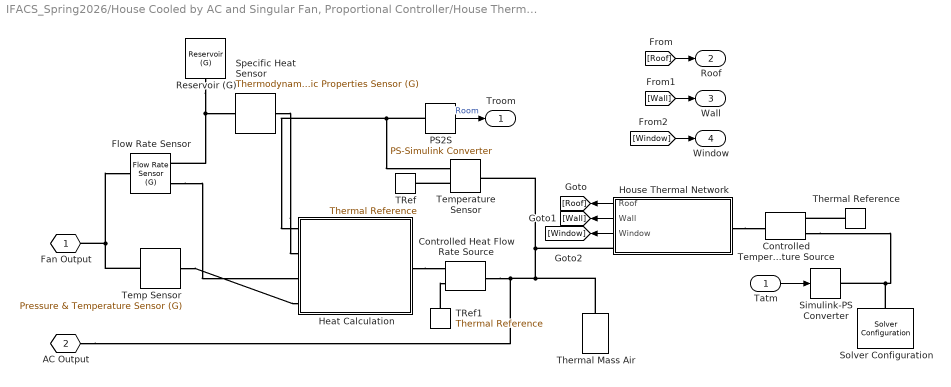
== system IFACS_Spring2026/House Cooled by AC and Singular Fan, Proportional Controller/House Thermal Network ==
  Tatm : Inport
  Controlled Temperature Source : fl_lib/Thermal/Thermal Sources/Controlled Temperature Source
  Controlled Heat Flow Rate Source : fl_lib/Thermal/Thermal Sources/Controlled Heat Flow Rate Source
  Flow Rate Sensor : fl_lib/Gas/Sensors/Flow Rate Sensor (G)  mass_flow_measure=true  volumetric_flow_measure=false  volumetric_flow_conditions=foundation.enum.volumetric_flow_conditions.actual  p_std=0.101325 MPa  T_std=20 degC  energy_flow_measure=false
      settings: InternalSimscapePortConfiguration="{\"Bottom\":[],\"Left\":[{\"id\":\"A\",\"label\":\"A\",\"type\":\"foundation.gas.gas\"}],\"Right\":[{\"id\":\"B\",\"label\":\"B\",\"type\":\"foundation.gas.gas\"},{\"id\":\"M\",\"label\":\"M\",\"type\":\"output\"}],\"Top\":[]}"
  Heat Calculation : Subsystem
  House Thermal Network : Subsystem  Tag=PublishSubsystem  mask(House Thermal Network){area_roof=2 * house_L * house_W / (2*cosd(roof_pitch)), thickness_roof=0.2, rho_roof=32, cp_roof=835, k_roof=0.038, hc_roof_interior=12, hc_roof_exterior=38, T_init_roof=TinIC, area_wall=2 * (house_L + house_W) * house_H, thickness_wall=0.2, rho_wall=1920, cp_wall=835, k_wall=0.038, hc_wall_interior=24, hc_wall_exterior=34, T_init_wall=TinIC, area_wall_inside=(house_L + 2 * house_W) * house_H + 2 * house_L * house_W, thickness_wall_inside=0.15, rho_wall_inside=10, cp_wall_inside=1000, k_wall_inside=0.2, hc_wall_inside_interior=24, T_init_wall_inside=TinIC, area_window=12, thickness_window=0.01, rho_window=2700, cp_window=840, k_window=0.78, hc_window_interior=25, hc_window_exterior=32, T_init_window=TinIC, area_furniture=300, M_furniture=3000, cp_furniture=2000, hc_furniture_interior=18, T_init_furniture=TinIC}
      mask prompts: area_roof "Total area (m^2)"; thickness_roof "Average thickness (m)"; rho_roof "Average density (kg/m^3)"; cp_roof "Average specific heat (J/kg/K)"; k_roof "Average conductivity (W/m/K)"; hc_roof_interior "Interior heat transfer coefficient (W/m^2/K)"; hc_roof_exterior "Exterior heat transfer coefficient (W/m^2/K)"; T_init_roof "Initial temperature (degC)"; area_wall "Total area (m^2)"; thickness_wall "Average thickness (m)"; rho_wall "Average density (kg/m^3)"; cp_wall "Average specific heat (J/kg/K)"; k_wall "Average conductivity (W/m/K)"; hc_wall_interior "Interior heat transfer coefficient (W/m^2/K)"; hc_wall_exterior "Exterior heat transfer coefficient (W/m^2/K)"; T_init_wall "Initial temperature (degC)"; area_wall_inside "Total area (m^2)"; thickness_wall_inside "Average thickness (m)"; rho_wall_inside "Average density (kg/m^3)"; cp_wall_inside "Average specific heat (J/kg/K)"; k_wall_inside "Average conductivity (W/m/K)"; hc_wall_inside_interior "Interior heat transfer coefficient (W/m^2/K)"; T_init_wall_inside "Initial temperature (degC)"; area_window "Total area (m^2)"; thickness_window "Average thickness (m)"; rho_window "Average density (kg/m^3)"; cp_window "Average specific heat (J/kg/K)"; k_window "Average conductivity (W/m/K)"; hc_window_interior "Interior heat transfer coefficient (W/m^2/K)"; hc_window_exterior "Exterior heat transfer coefficient (W/m^2/K)"; T_init_window "Initial temperature (degC)"; area_furniture "Total surface area (m^2)"; M_furniture "Total mass (kg)"; cp_furniture "Average specific heat (J/kg/K)"; hc_furniture_interior "Interior heat transfer coefficient (W/m^2/K)"; T_init_furniture "Initial temperature (degC)"
      mask help: This subsystem models heat transfer between the air in the interior of the house and the external environment.
      mask DialogControl TabRoof Prompt: Roof
      mask DialogControl TabWall Prompt: Exterior Walls
      mask DialogControl TabWallInside Prompt: Interior Walls
      mask DialogControl TabWindow Prompt: Windows
      mask DialogControl TabFurniture Prompt: Furniture
  PS2S : nesl_utility/PS-Simulink Converter  PhysicalDomain=network_engine_domain  SubClassName=ps_output  LeftPortType=input  RightPortType=output  PseudoPeriodic=off  Frequencies=[]  VectorFormat=1-D array  Unit=degC  AffineConversion=on
  Reservoir (G) : fl_lib/Gas/Elements/Reservoir (G)  pressure_spec=foundation.enum.pressure_spec.atmospheric  reservoir_pressure=0.101325 MPa  reservoir_temperature=293.15 K  area_A=0.01 m^2
  Simulink-PS Converter : nesl_utility/Simulink-PS Converter  PhysicalDomain=network_engine_domain  SubClassName=ps_input  LeftPortType=input  RightPortType=output  PseudoPeriodic=off  Frequencies=[]  NoiseDistribution=none  NoiseParameters=[]  Unit=degC  AffineConversion=on  FilteringAndDerivatives=zero  SimscapeFilterOrder=1  InputFilterTimeConstant=.001  UdotUserProvided=0
  Solver Configuration : nesl_utility/Solver Configuration  PhysicalDomain=network_engine_domain  SubClassName=solver  LeftPortType=input  RightPortType=generic  Tones=[]  Harmonics=[]  SimulateNoise=off  Profile=off  UseLocalSampling=off  EnableSwitchedLinearOptims=on  FrequencyDomain=off  UseCCode=off  RelTol=0.001  AbsTol=1e-06  MinStep=1e-09  ToWorkspace=off  RevertToSquareIcSolve=off  NumHomotopyIterations=100  PhasorMode=off  PhasorModeNumHarmonics=1  ConsistencySolver=NEWTON_XTOL_AFTER_FTOL  IndexReductionMethod=DerivativeReplacement  DoDC=off  ResidualTolerance=1e-9  ConsistencyTolSource=GLOBAL  ConsistencyAbsTol=0.001  ConsistencyRelTol=0.001  ConsistencyTolFactor=0.001  UseLocalSolver=off  LocalSolverChoice=NE_BACKWARD_EULER_ADVANCER  ResolveIndetEquations=on  FunctionEvalNumThread=1  LocalSolverSampleTime=1  DoFixedCost=off  MaxNonlinIter=3  MaxModeIter=2  ComputeImpulses=off  ImpulseIterations=2  LinearAlgebra=auto  LinearAlgebraNumThread=0  EquationFormulation=NE_TIME_EF  DelaysMemoryBudget=1024  AutomaticFiltering=on  FilteringTimeConstant=0.001  PartitionStorageMethod=AS_NEEDED  PartitionMemoryBudget=1024  PartitionMethod=FAST  MultibodyUseLocalSolver=off  MultibodyLocalSolverChoice=ODE1  MultibodyLocalSolverSampleTime=0.001
  Specific Heat Sensor : fl_lib/Gas/Sensors/Thermodynamic Properties Sensor (G)  enthalpy=false  density=false  specific_heat=true  entropy=false  s_std=3.8635 kJ/(K*kg)  p_std=0.101325 MPa  T_std=293.15 K
      settings: InternalSimscapePortConfiguration="{\"Bottom\":[{\"id\":\"CP\",\"label\":\"cp\",\"type\":\"output\"}],\"Left\":[{\"id\":\"A\",\"label\":\"A\",\"type\":\"foundation.gas.gas\"}],\"Right\":[],\"Top\":[]}"
  TRef : fl_lib/Thermal/Thermal Elements/Thermal Reference
  TRef1 : fl_lib/Thermal/Thermal Elements/Thermal Reference
  Temp Sensor : fl_lib/Gas/Sensors/Pressure & Temperature Sensor (G)  reference=foundation.enum.MeasurementReference.absolute  pressure=false  pressure_spec=foundation.enum.PressureMeasementSpec.Absolute  temperature=true
      settings: InternalSimscapePortConfiguration="{\"Bottom\":[{\"id\":\"T\",\"label\":\"T\",\"type\":\"output\"}],\"Left\":[{\"id\":\"A\",\"label\":\"A\",\"type\":\"foundation.gas.gas\"}],\"Right\":[],\"Top\":[]}"
  Temperature Sensor : fl_lib/Thermal/Thermal Sensors/Temperature Sensor  temperature_measure=foundation.enum.MeasurementReference.difference
  Thermal Mass Air : fl_lib/Thermal/Thermal Elements/Thermal Mass  mass_type=foundation.enum.constant_variable.constant  mass=1600 kg  sp_heat=c_air J/kg/K  mass_min=1e-6 kg  num_ports=foundation.enum.numPorts2.one  m_specify=off  m_priority=High  m=1 kg  m_nominal_specify=off  m_nominal_value=1  m_nominal_unit=kg  T_specify=on  T_priority=High  T=TinIC degC  T_nominal_specify=off  T_nominal_value=1  T_nominal_unit=K  Q_specify=off  Q_priority=None  Q=0 W  Q_nominal_specify=off  Q_nominal_value=1  Q_nominal_unit=W
  Thermal Reference : fl_lib/Thermal/Thermal Elements/Thermal Reference
  Fan Output : PMIOPort  Tag=PMCPort  Side=Left
  AC Output : PMIOPort  Tag=PMCPort  Port=2  Side=Left
  Troom : Outport  VectorParamsAs1DForOutWhenUnconnected=off
  Roof : Outport  Port=2  VectorParamsAs1DForOutWhenUnconnected=off
  Wall : Outport  Port=3  VectorParamsAs1DForOutWhenUnconnected=off
  Window : Outport  Port=4  VectorParamsAs1DForOutWhenUnconnected=off
  wires:
  Tatm/1 -> Simulink-PS Converter/1
  House Thermal Network/1(Roof) -> [Roof]
  [Roof] -> Roof/1
  House Thermal Network/2(Wall) -> [Wall]
  [Wall] -> Wall/1
  House Thermal Network/3(Window) -> [Window]
  [Window] -> Window/1
  PS2S/1 -> Troom/1  "Room"
  connections:
  Thermal Reference/LConn1 -- Controlled Temperature Source/RConn2
  Controlled Temperature Source/RConn1 -- Solver Configuration/RConn1 -- Simulink-PS Converter/RConn1
  TRef1/LConn1 -- Controlled Heat Flow Rate Source/RConn2
  Temp Sensor/LConn1 -- Flow Rate Sensor/LConn1 -- Fan Output/RConn1
  Reservoir (G)/LConn1 -- Flow Rate Sensor/RConn1 -- Specific Heat Sensor/LConn1
  Temperature Sensor/LConn1 -- House Thermal Network/RConn1 -- Controlled Heat Flow Rate Source/LConn1 -- AC Output/RConn1 -- Thermal Mass Air/LConn1
  Temperature Sensor/RConn1 -- TRef/LConn1
  PS2S/LConn1 -- Heat Calculation/LConn1 -- Temperature Sensor/RConn2
  Specific Heat Sensor/RConn1 -- Heat Calculation/LConn2
  Flow Rate Sensor/RConn2 -- Heat Calculation/LConn3
  Temp Sensor/RConn1 -- Heat Calculation/LConn4
  Heat Calculation/RConn1 -- Controlled Heat Flow Rate Source/RConn1
  House Thermal Network/LConn1 -- Controlled Temperature Source/LConn1

== system IFACS_Spring2026/House Cooled by Singular Fan, Bang Bang Controller/Fan Cost Calculation ==
  Fanpwr : Inport
  Electricity Cost (per kWh) : Gain  Gain=.15
  Fan Wattage : Gain  Gain=68.9/(1000*3600)
  Integrator : Integrator
  Fan Electrical Cost : Outport
  wires:
  Electricity Cost (per kWh)/1 -> Fan Electrical Cost/1  "Fan Electricity Cost"
  Integrator/1 -> Fan Wattage/1
  Fan Wattage/1 -> Electricity Cost (per kWh)/1
  Fanpwr/1 -> Integrator/1

== system IFACS_Spring2026/House Cooled by Singular Fan, Bang Bang Controller/Fan Parameters ==
  note: Current Fan used in Simulation
      | https://www.homedepot.com/p/KIWDZFU-720-CFM-Wall-Mounted-Ventilation-Fan-for-Home-Garage-and-Office-Use-423D22SA17036/335970250?MERCH=REC-_-brand_based_collection-_-335970202-_-3-_-n/a-_-n/a-_-n/a-_-n/a-_-n/a
  Tmin : Inport
  Troom : Inport  Port=2
  Tenv : Inport  Port=3
  Fan Activation : Subsystem
  House Fan : Subsystem
  Fan Output : PMIOPort  Side=Right
  Fan Total Power : Outport
  wires:
  Fan Activation/1(Fan Activation) -> House Fan/1(Fan Activation)
  Tmin/1 -> Fan Activation/1(Tmin)
  Tenv/1 -> Fan Activation/3(Tenv), House Fan/2(Tenv)
  House Fan/1(Fan Total Power) -> Fan Total Power/1
  Troom/1 -> Fan Activation/2(Room)
  connections:
  Fan Output/RConn1 -- House Fan/RConn1
